simulink model "PID"  (R2022b)
settings: Solver=VariableStepAuto  StartTime=0.0  StopTime=10.0  RelTol=1e-3
model workspace (MAT data in the model file):
  Cw = Simulink.Parameter
  Cw.Value = 4.19
  Cw.DataType = 'auto'
  Cw.Complexity = 'real'
  Cw.Dimensions = [1 1]
  Kp = 5
  Tn = 3
  k = Simulink.Parameter
  k.Value = 2
  k.DataType = 'auto'
  k.Complexity = 'real'
  k.Dimensions = [1 1]
  mw = Simulink.Parameter
  mw.Value = 0.05
  mw.DataType = 'auto'
  mw.Complexity = 'real'
  mw.Dimensions = [1 1]
settings Model: ParameterArgumentNames=Kp,Tn  Creator=fgewi  LastModifiedBy=fgewi

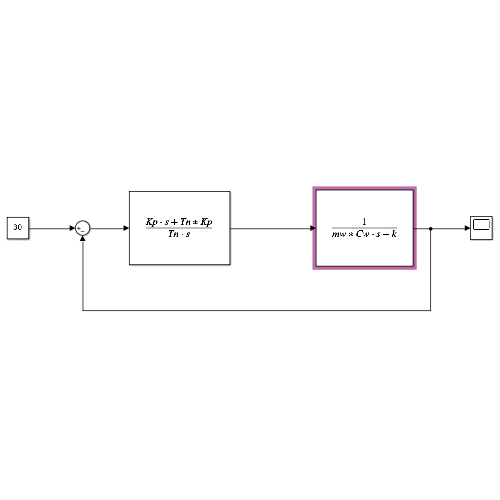
[thumbnail: Simulink's stored preview of the top-level diagram]
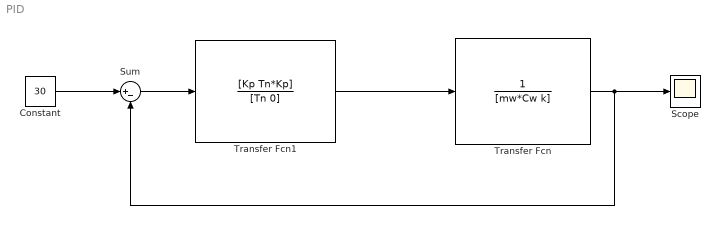
== system PID ==
  Constant : Constant  Value=30
  Scope : Scope
  Sum : Sum  Inputs=|+-
  Transfer Fcn : TransferFcn  Denominator=[mw*Cw k]
  Transfer Fcn1 : TransferFcn  Numerator=[Kp Tn*Kp]  Denominator=[Tn 0]  ParameterTunability=Unconstrained
  wires:
  Transfer Fcn1/1 -> Transfer Fcn/1
  Sum/1 -> Transfer Fcn1/1
  Transfer Fcn/1 -> Sum/2, Scope/1
  Constant/1 -> Sum/1
